simulink model "CruiseCntrl"  (R2020b)
settings: Solver=VariableStepAuto  StartTime=0.0  StopTime=10.0  RelTol=1e-3
values from neighbouring files (symbols this model uses):
  b = 50.0    [Cruise_DataDictionary.sldd]
  Ki = 40.0    [Cruise_DataDictionary.sldd]
  Kp = 800.0    [Cruise_DataDictionary.sldd]
  m = 1000.0    [Cruise_DataDictionary.sldd]
settings Model: DataDictionary=Cruise_DataDictionary.sldd  Creator=Sourav Kumar  LastModifiedBy=Sourav Kumar

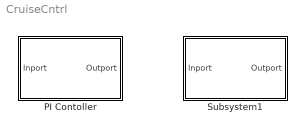
== system CruiseCntrl ==
  PI Contoller : Subsystem
  Subsystem1 : Subsystem

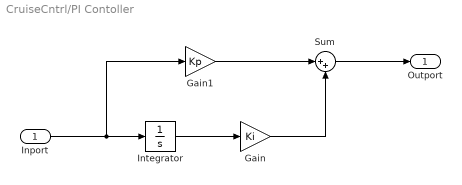
== system CruiseCntrl/PI Contoller ==
  Inport : Inport
  Gain : Gain  Gain=Ki
  Gain1 : Gain  Gain=Kp
  Integrator : Integrator
  Sum : Sum  Inputs=|++
  Outport : Outport
  wires:
  Gain/1 -> Sum/2
  Inport/1 -> Gain1/1, Integrator/1
  Integrator/1 -> Gain/1
  Sum/1 -> Outport/1
  Gain1/1 -> Sum/1

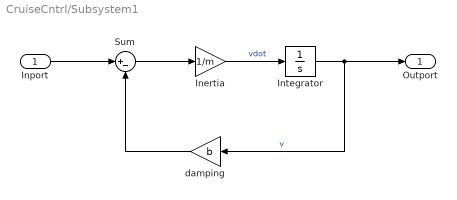
== system CruiseCntrl/Subsystem1 ==
  Inport : Inport
  Inertia : Gain  Gain=1/m
  Integrator : Integrator
  Sum : Sum  Inputs=|+-
  damping : Gain  Gain=b
  Outport : Outport
  wires:
  Inport/1 -> Sum/1
  Inertia/1 -> Integrator/1  "vdot"
  Sum/1 -> Inertia/1
  Integrator/1 -> Outport/1, damping/1  "v"
  damping/1 -> Sum/2
